simulink model "MOD_ANA_MAKRIS"  (R2017b)
settings: Solver=FixedStepAuto  StartTime=0.0  StopTime=4.25  FixedStep=0.01  RelTol=1e-3  EnableMultiTasking=on
undefined symbols (not defined in the file or in its folder): m, sigma, wo
settings Model: ExtModeTrigDuration=2  Creator=ferca  LastModifiedBy=Dr. Candia
settings DataIOCC: ReturnWorkspaceOutputs=on
settings OptimizationCC: EnhancedBackFolding=on  PassReuseOutputArgsThreshold=0  MaxStackSize=64  OptimizeBlockOrder=speed  DifferentSizesBufferReuse=on
settings DebuggingCC: ParameterTunabilityLossMsg=error
settings HardwareCC: ProdBitPerInt=16  ProdBitPerPointer=16  ProdBitPerSizeT=16  ProdBitPerPtrDiffT=16  ProdLargestAtomicFloat=None  ProdWordSize=8  ProdHWDeviceType=Atmel->AVR
settings SFSimCC: SimUseLocalCustomCode=on  MATLABDynamicMemAlloc=off
settings RTWCC: SystemTargetFile=ert.tlc  HardwareBoard=Arduino Uno  TLCOptions=-aInlineSetEventsForThisBaseRateFcn=TLC_FALSE -aSuppressMultiTaskScheduler=TLC_FALSE -aRateBasedStepFcn=1  TemplateMakefile=ert_default_tmf  GenerateReport=on  RTWUseLocalCustomCode=on  Toolchain=Arduino AVR  BuildConfiguration=Faster Runs  LaunchReport=on
settings CodeAppCC: ForceParamTrailComments=on  OperatorAnnotations=on  MangleLength=10
settings ERTTargetCC: ERTCustomFileBanners=off  SupportContinuousTime=on  SupportNonInlinedSFcns=on  RemoveResetFunc=off  SupportVariableSizeSignals=on  ModelStepFunctionPrototypeControlCompliant=off  ExtModeStaticAllocSize=2048

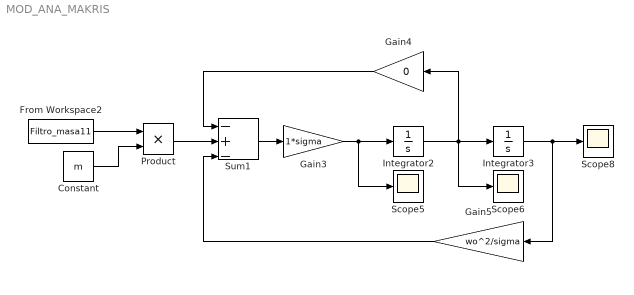
== system MOD_ANA_MAKRIS ==
  Constant : Constant  Value=m
  From Workspace2 : FromWorkspace  VariableName=Filtro_masa11  SampleTime=0
  Gain3 : Gain  Gain=1*sigma
  Gain4 : Gain  Gain=0
  Gain5 : Gain  Gain=wo^2/sigma
  Integrator2 : Integrator
  Integrator3 : Integrator
  Product : Product
  Scope5 : Scope
  Scope6 : Scope
  Scope8 : Scope
  Sum1 : Sum  Inputs=|-|+|-
  wires:
  Gain5/1 -> Sum1/3
  Sum1/1 -> Gain3/1
  Integrator2/1 -> Gain4/1, Scope6/1, Integrator3/1
  Gain3/1 -> Scope5/1, Integrator2/1
  Integrator3/1 -> Scope8/1, Gain5/1
  Gain4/1 -> Sum1/1
  Constant/1 -> Product/2
  Product/1 -> Sum1/2
  From Workspace2/1 -> Product/1
